simulink model "spline_sim"  (R2019b)
settings: Solver=VariableStepAuto  StartTime=0.0  StopTime=2  FixedStep=0.006  RelTol=1e-3
values from neighbouring files (symbols this model uses):
  Econst = zeros(2,1)    [Main.m]    (also in model_parameters.m)
  L = 2.0    (= 2)    [Main.m]    (also in model_parameters.m)
  Mld = setModel(Mld,sectionType,R1,R2,E,Bt,V,rho,FApos,FAneg,FBpos,FBneg,du,L,m,p,nd,nC)    [Main.m]    (also in model_parameters.m)
  Yinit = vec2mat(Y(end,:),Mld.nControlPoints)'    [matlab_simulation.m]
settings Model: SimulationMode=accelerator  Creator=luca  LastModifiedBy=luca
settings OptimizationCC: DefaultParameterBehavior=Inlined  UseDivisionForNetSlopeComputation=on  GainParamInheritBuiltInType=on  UseFloatMulNetSlope=on  InlineInvariantSignals=on  PassReuseOutputArgsThreshold=0  EfficientFloat2IntCast=on  OptimizeBlockOrder=speed  DifferentSizesBufferReuse=on
settings DebuggingCC: ParameterTunabilityLossMsg=error
settings HardwareCC: ProdBitPerLong=64  ProdLongLongMode=on  ProdHWDeviceType=Intel->x86-64 (Linux 64)  TargetBitPerLong=64  TargetBitPerPointer=64  TargetBitPerSizeT=64  TargetBitPerPtrDiffT=64  TargetLongLongMode=on  TargetIntDivRoundTo=Zero  TargetEndianess=LittleEndian  TargetWordSize=64  TargetHWDeviceType=MATLAB Host  ProdEqTarget=off
settings SFSimCC: MATLABDynamicMemAlloc=off  CustomCodeUndefinedFunction=UseInterfaceOnly
settings RTWCC: Description=Rapid Simulation Target  SystemTargetFile=rsim.tlc  TemplateMakefile=rsim_default_tmf  GenerateReport=on  BuildConfiguration=Faster Runs  LaunchReport=on  TargetLang=C++
settings CodeAppCC: ForceParamTrailComments=on  OperatorAnnotations=on
settings TargetCC: TargetLangStandard=C++03 (ISO)  ParMdlRefBuildCompliant=on  ConcurrentExecutionCompliant=on  GeneratePreprocessorConditionals=Use local settings  MatFileLogging=on  PreserveStateflowLocalDataDimensions=off

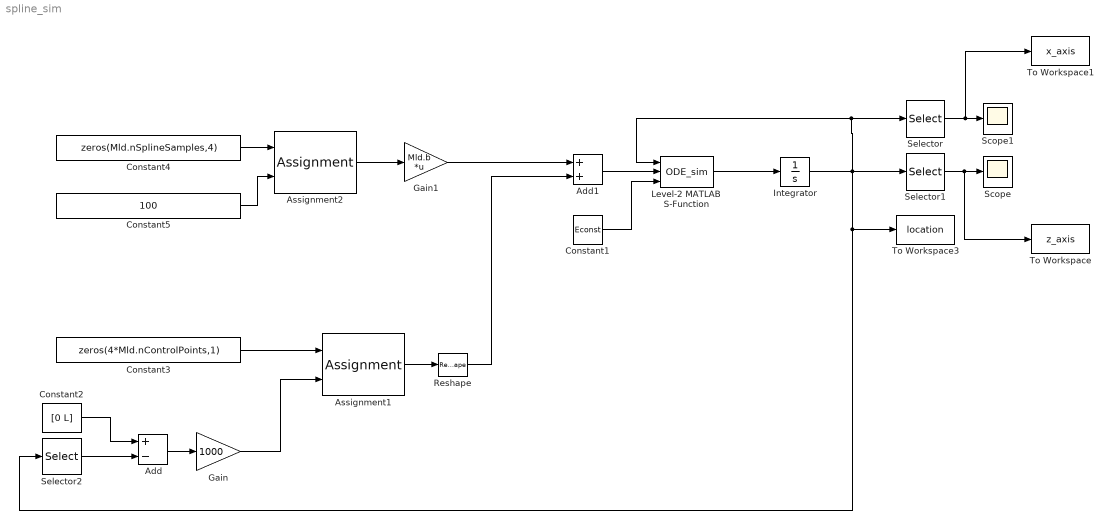
== system spline_sim ==
  Add : Sum  Inputs=+-
  Add1 : Sum
  Assignment1 : Assignment  DiagnosticForDimensions=Warning  IndexOptions=Index vector (dialog)  Indices=[1 Mld.nControlPoints]  OutputSizes=1
  Assignment2 : Assignment  NumberOfDimensions=2  DiagnosticForDimensions=Warning  IndexOptions=Index vector (dialog),Index vector (dialog)  Indices=[35],3  OutputSizes=1,1
  Constant1 : Constant  Value=Econst
  Constant2 : Constant  Value=[0 L]
  Constant3 : Constant  Value=zeros(4*Mld.nControlPoints,1)
  Constant4 : Constant  Value=zeros(Mld.nSplineSamples,4)
  Constant5 : Constant  Value=100
  Gain : Gain  Gain=1000
  Gain1 : Gain  Gain=Mld.b  Multiplication=Matrix(K*u)
  Integrator : Integrator  InitialCondition=Yinit(:)
  Level-2 MATLAB S-Function : M-S-Function  FunctionName=ODE_sim  Parameters=Mld
  Reshape : Reshape  OutputDimensionality=Customize  OutputDimensions=[Mld.nControlPoints,4]
  Scope : Scope
  Scope1 : Scope
  Selector : Selector  InputPortWidth=8*Mld.nControlPoints  IndexOptions=Index vector (dialog)  Indices=[1:Mld.nControlPoints]  OutputSizes=1
  Selector1 : Selector  InputPortWidth=8*Mld.nControlPoints  IndexOptions=Index vector (dialog)  Indices=[Mld.nControlPoints*2+1:Mld.nControlPoints*3]  OutputSizes=1
  Selector2 : Selector  InputPortWidth=8*Mld.nControlPoints  IndexOptions=Index vector (dialog)  Indices=[1 Mld.nControlPoints]  OutputSizes=1
  To Workspace : ToWorkspace  VariableName=z_axis  SampleTime=-1
  To Workspace1 : ToWorkspace  VariableName=x_axis  SampleTime=-1
  To Workspace3 : ToWorkspace  VariableName=location  SampleTime=-1
      settings: Save2DSignal=2-D array (concatenate along first dimension)
  wires:
  Level-2 MATLAB S-Function/1 -> Integrator/1
  Integrator/1 -> Selector/1, Level-2 MATLAB S-Function/1, Selector2/1, To Workspace3/1, Selector1/1
  Constant1/1 -> Level-2 MATLAB S-Function/3
  Selector/1 -> To Workspace1/1, Scope1/1
  Selector1/1 -> To Workspace/1, Scope/1
  Constant2/1 -> Add/1
  Selector2/1 -> Add/2
  Add/1 -> Gain/1
  Gain/1 -> Assignment1/2
  Assignment1/1 -> Reshape/1
  Constant3/1 -> Assignment1/1
  Reshape/1 -> Add1/2
  Constant4/1 -> Assignment2/1
  Constant5/1 -> Assignment2/2
  Add1/1 -> Level-2 MATLAB S-Function/2
  Assignment2/1 -> Gain1/1
  Gain1/1 -> Add1/1
